simulink model "Balance_Control"  (R2020b)
settings: Solver=VariableStepAuto  StartTime=0.0  StopTime=10.0  RelTol=1e-3
values from neighbouring files (symbols this model uses):
  K = lqr( A, B(:,2), Q, R )    [Active_suspension_open_loop_setup.m]
  ks = 900    [Active_suspension_open_loop_setup.m]
settings Model: Creator=admin  LastModifiedBy=admin

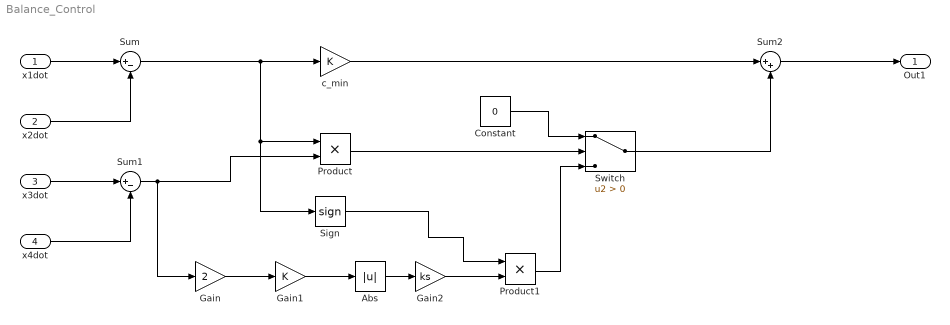
== system Balance_Control ==
  x1dot : Inport
  x2dot : Inport  Port=2
  x3dot : Inport  Port=3
  x4dot : Inport  Port=4
  Abs : Abs
  Constant : Constant  Value=0
  Gain : Gain  Gain=2
  Gain1 : Gain  Gain=K
  Gain2 : Gain  Gain=ks
  Product : Product
  Product1 : Product
  Sign : Signum
  Sum : Sum  Inputs=|+-
  Sum1 : Sum  Inputs=|+-
  Sum2 : Sum  Inputs=|++
  Switch : Switch  Criteria=u2 > Threshold
  c_min : Gain  Gain=K
  Out1 : Outport
  wires:
  x1dot/1 -> Sum/1
  x2dot/1 -> Sum/2
  x3dot/1 -> Sum1/1
  x4dot/1 -> Sum1/2
  Sum/1 -> Sign/1, Product/1, c_min/1
  c_min/1 -> Sum2/1
  Switch/1 -> Sum2/2
  Sum2/1 -> Out1/1
  Constant/1 -> Switch/1
  Product/1 -> Switch/2
  Sum1/1 -> Gain/1, Product/2
  Sign/1 -> Product1/1
  Gain/1 -> Gain1/1
  Gain1/1 -> Abs/1
  Abs/1 -> Gain2/1
  Gain2/1 -> Product1/2
  Product1/1 -> Switch/3
